simulink model "W02_B_second_order"  (R2024b)
settings: Solver=ode4  StartTime=0  StopTime=T_final  FixedStep=h  RelTol=1e-3
values from neighbouring files (symbols this model uses):
  t_step = 1    [W02_0_setup.m]
  wn = 2    [W02_0_setup.m]    (also in W02_C_proportional_only.m = sqrt(k + Kp); W02_E_integral_and_derivative.m = sqrt(V.K_u*V.Ki_d/te))
  y_step = 1    [W02_0_setup.m]
  zeta = 0.5    [W02_0_setup.m]    (also in W02_I_tuning_by_hand.m = -L/sqrt(pi^2 + L^2))
settings Model: Creator=admin  LastModifiedBy=admin
settings DataIOCC: ReturnWorkspaceOutputs=off

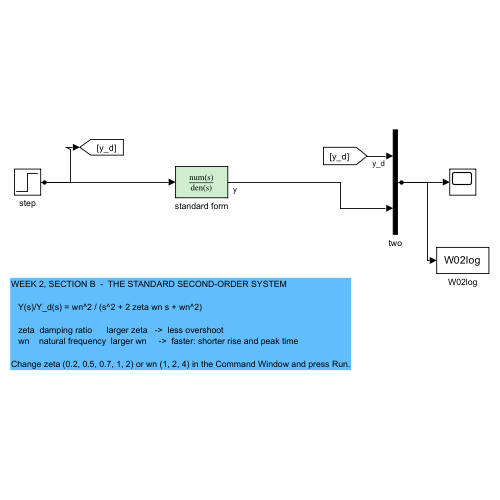
[thumbnail: Simulink's stored preview of the top-level diagram]
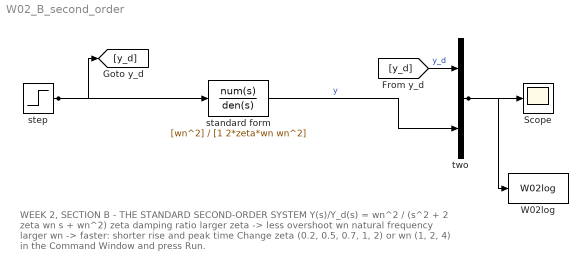
== system W02_B_second_order ==
  note: WEEK 2, SECTION B  -  THE STANDARD SECOND-ORDER SYSTEM
      |
      |    Y(s)/Y_d(s) = wn^2 / (s^2 + 2 zeta wn s + wn^2)
      |
      |    zeta  damping ratio      larger zeta   ->  less overshoot
      |    wn    natural frequency  larger wn     ->  faster: shorter rise and peak time
      |
      | Change zeta (0.2, 0.5, 0.7, 1, 2) or wn (1, 2, 4) in the Command Window and press Run.
  Scope : Scope
  W02log : ToWorkspace  VariableName=W02log  SaveFormat=Structure With Time  SampleTime=-1
  standard form : TransferFcn  Numerator=[wn^2]  Denominator=[1 2*zeta*wn wn^2]
  step : Step  Time=t_step  After=y_step  SampleTime=0
  two : Mux  Inputs=2
  wires:
  step/1 -> standard form/1, [y_d]
  [y_d] -> two/1  "y_d"
  standard form/1 -> two/2  "y"
  two/1 -> Scope/1, W02log/1
